simulink library "Lib_Solve_IterNRSolverJC_TMATS"  (R2013b)
settings: Solver=ode45  StartTime=0.0  StopTime=10.0  RelTol=1e-3
libraries: Lib_NM_JacobianCalc_TMATS x1, Lib_NM_NewtonRaphsonSolver_TMATS x1
Description:
  | Thomas Modules
settings Model: Creator=jwchapm2  LastModifiedBy=jwchapm2

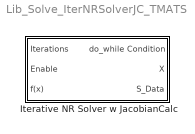
== system Lib_Solve_IterNRSolverJC_TMATS ==
  Iterative NR Solver w JacobianCalc : Subsystem  mask(T-MATS: Iterative NR Solver w Jacobian Calc Library Block){SJac_Per_M=[0.01; 0.05; 0.05], SNR_IC_M=[1 2 3], SNR_DX_M=5, SJacobianAttempts_M=20, Cond_Limits_M=0.01}
      mask prompts: SJac_Per_M "SJac_Per_M - Jacobian Perturbation size (frac) (nx1)"; SNR_IC_M "SNR_IC_M - Newton Raphson Initial Conditions (nx1)"; SNR_DX_M "SNR_DX_M - Newton Raphson delta x limiter (%) (1x1)"; SJacobianAttempts_M "SJacobianAttempts_M - Newton Raphson attempts before the Jacobian recalculation (1x1)"; Cond_Limits_M "Cond_Limits_M - Iteration Conditions Limits (nx1 or 1x1)"
      mask help:
      | The Iterative Newton Raphson Solver with Jacobian Calculator block will
      | supply the inputs to iteratively drive the outputs of a system to zero.
      |
      | This will be performed in three steps.
      | 1) Jabobian calculator sends Perturbations to the plant then calculates the plant
      | Jacboian based on the system response
      | 2) The Newton Raphson will use the inverse of the Jacobian to iteratively step the
      | system toward solution.
      | 3) Once the solution has satisfied the conditions the Newton Raphson is shut off.
      |
      | This module is designed for dynamic systems and should be paired with
      | a "do... while" block in Simulink. The "do...while" block and this module
      | should both be located in the same subsystem as the plant that is to be solved for.
      mask Help: web(which('Solver_TMATS_INRSwJC.html'),'-helpbrowser')

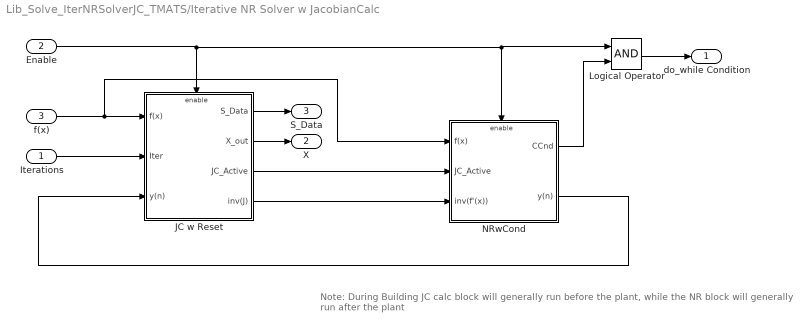
== system Lib_Solve_IterNRSolverJC_TMATS/Iterative NR Solver w JacobianCalc ==
  note: Note: During Building JC calc block will generally run before the plant, while the NR block will generally run after the plant
  Iterations : Inport
  Enable : Inport  Port=2
  f(x) : Inport  Port=3
  JC w Reset : Subsystem
  Logical Operator : Logic  AllPortsSameDT=off  OutDataTypeStr=boolean
  NRwCond : Subsystem
  do_while Condition : Outport
  X : Outport  Port=2
  S_Data : Outport  Port=3
  wires:
  f(x)/1 -> NRwCond/1(f(x)), JC w Reset/1(f(x))
  NRwCond/1(CCnd) -> Logical Operator/2
  Iterations/1 -> JC w Reset/2(Iter)
  NRwCond/2(y(n)) -> JC w Reset/3(y(n))
  JC w Reset/1(S_Data) -> S_Data/1
  JC w Reset/2(X_out) -> X/1
  JC w Reset/3(JC_Active) -> NRwCond/2(JC_Active)
  JC w Reset/4(inv(J)) -> NRwCond/3(inv(f'(x)))
  Enable/1 -> NRwCond/Enable, Logical Operator/1, JC w Reset/Enable
  Logical Operator/1 -> do_while Condition/1

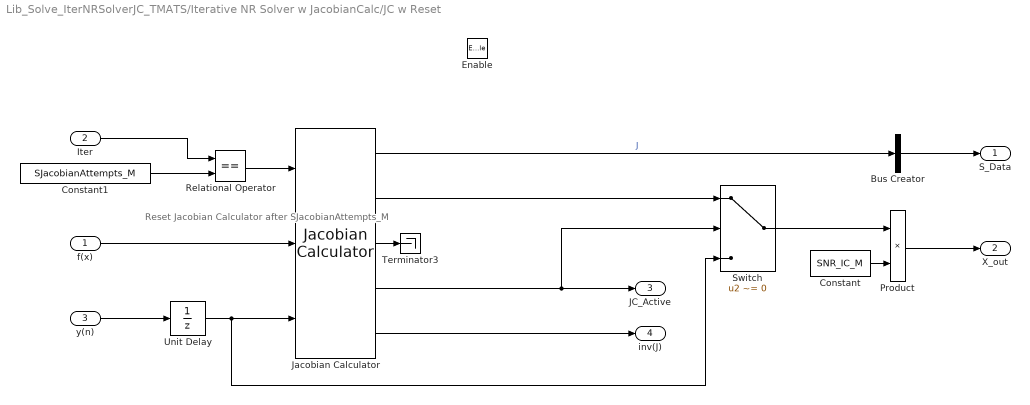
== system Lib_Solve_IterNRSolverJC_TMATS/Iterative NR Solver w JacobianCalc/JC w Reset ==
  note: Reset Jacobian Calculator after SJacobianAttempts_M
  f(x) : Inport
  Iter : Inport  Port=2
  y(n) : Inport  Port=3
  Enable : EnablePort
  Bus Creator : BusCreator  Inputs=1
  Constant : Constant  Value=SNR_IC_M
  Constant1 : Constant  Value=SJacobianAttempts_M  OutDataTypeStr=uint32
  Jacobian Calculator : Lib_NM_JacobianCalc_TMATS/Jacobian Calculator  N_Per_M=SJac_Per_M
  Product : Product  RndMeth=Zero
  Relational Operator : RelationalOperator  Operator===  OutDataTypeStr=boolean
  Switch : Switch  Criteria=u2 ~= 0  Threshold=1
  Terminator3 : Terminator
  Unit Delay : UnitDelay  InitialCondition=ones(length(SNR_IC_M),1)  SampleTime=-1
  S_Data : Outport
  X_out : Outport  Port=2
  JC_Active : Outport  Port=3
  inv(J) : Outport  Port=4
  wires:
  f(x)/1 -> Jacobian Calculator/2
  Jacobian Calculator/5 -> inv(J)/1
  Unit Delay/1 -> Switch/3, Jacobian Calculator/3
  y(n)/1 -> Unit Delay/1
  Jacobian Calculator/1 -> Bus Creator/1  "J"
  Constant/1 -> Product/2
  Relational Operator/1 -> Jacobian Calculator/1
  Product/1 -> X_out/1
  Jacobian Calculator/2 -> Switch/1
  Switch/1 -> Product/1
  Jacobian Calculator/4 -> JC_Active/1, Switch/2
  Constant1/1 -> Relational Operator/2
  Iter/1 -> Relational Operator/1
  Bus Creator/1 -> S_Data/1
  Jacobian Calculator/3 -> Terminator3/1

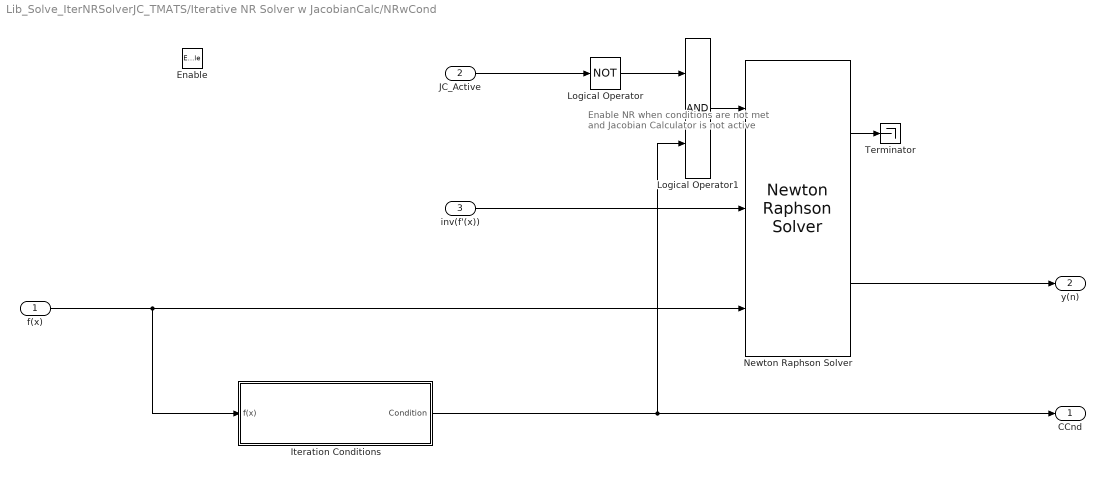
== system Lib_Solve_IterNRSolverJC_TMATS/Iterative NR Solver w JacobianCalc/NRwCond ==
  note: Enable NR when conditions are not met
      | and Jacobian Calculator is not active
  f(x) : Inport
  JC_Active : Inport  Port=2
  inv(f'(x)) : Inport  Port=3
  Enable : EnablePort
  Iteration Conditions : Subsystem
  Logical Operator : Logic  Operator=NOT  AllPortsSameDT=off  OutDataTypeStr=boolean
  Logical Operator1 : Logic  AllPortsSameDT=off  OutDataTypeStr=boolean
  Newton Raphson Solver : Lib_NM_NewtonRaphsonSolver_TMATS/Newton Raphson Solver  NR_IC_M=ones(length(SNR_IC_M),1)  NR_dx_Lim_M=SNR_DX_M
  Terminator : Terminator
  CCnd : Outport
  y(n) : Outport  Port=2
  wires:
  f(x)/1 -> Iteration Conditions/1(f(x)), Newton Raphson Solver/3
  JC_Active/1 -> Logical Operator/1
  Newton Raphson Solver/2 -> y(n)/1
  Newton Raphson Solver/1 -> Terminator/1
  inv(f'(x))/1 -> Newton Raphson Solver/2
  Logical Operator1/1 -> Newton Raphson Solver/1
  Logical Operator/1 -> Logical Operator1/1
  Iteration Conditions/1(Condition) -> Logical Operator1/2, CCnd/1

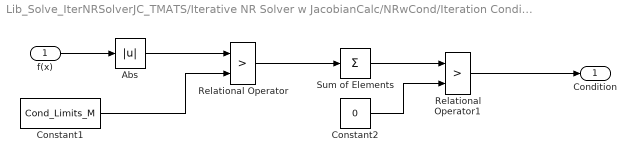
== system Lib_Solve_IterNRSolverJC_TMATS/Iterative NR Solver w JacobianCalc/NRwCond/Iteration Conditions ==
  f(x) : Inport
  Abs : Abs
  Constant1 : Constant  Value=Cond_Limits_M
  Constant2 : Constant  Value=0
  Relational Operator : RelationalOperator  Operator=>  OutDataTypeStr=boolean
  Relational Operator1 : RelationalOperator  Operator=>  OutDataTypeStr=boolean
  Sum of Elements : Sum  Inputs=+
  Condition : Outport
  wires:
  Relational Operator1/1 -> Condition/1
  Sum of Elements/1 -> Relational Operator1/1
  Constant2/1 -> Relational Operator1/2
  Relational Operator/1 -> Sum of Elements/1
  f(x)/1 -> Abs/1
  Constant1/1 -> Relational Operator/2
  Abs/1 -> Relational Operator/1
